simulink model "six_plus_six_AcmsteeringV10_main"  (R2014a)
settings: Solver=FixedStepDiscrete  StartTime=0.0  StopTime=10.0  FixedStep=0.0005  RelTol=1e-3
InitFcn:
  | Veh_Par_wxt
values from neighbouring files (symbols this model uses):
  acc_spdctl = [0 100]    [Veh_Par_wxt.m]
  ag_thr = ecucoder_cal(ag_thr)    [Veh_Par_wxt.m]
  B = 1.8    [Veh_Par_wxt.m]
  bra_em = 100    [Veh_Par_wxt.m]
  bra_pre_gz2 = 100/3    (= 33.3333333333)    [Veh_Par_wxt.m]
  bra_pre_gz34 = 10/3    (= 3.33333333333)    [Veh_Par_wxt.m]
  bra_pre_yd = 10/2    (= 5)    [Veh_Par_wxt.m]
  brakepre_dem_data = [0 1 2 3 4 5 6 7 8 9 10]    [Veh_Par_wxt.m]
  brakeTrq_dem_data = [0 125 251 376 502 627 753 878 1004 1129 1255]    [Veh_Par_wxt.m]
  bratrq_max = 4*1255    (= 5020)    [Veh_Par_wxt.m]
  eff_tran = 0.9    [Veh_Par_wxt.m]
  ESP_switch = ecucoder_cal(ESP_switch)    [Veh_Par_wxt.m]
  G = Mass*g    (= 15696)    [Veh_Par_wxt.m]
  kd1 = ecucoder_cal(kd1)    [Veh_Par_wxt.m]
  kd2 = 0    [Veh_Par_wxt.m]
  ki1 = ecucoder_cal(ki1)    [Veh_Par_wxt.m]
  ki2 = 1    [Veh_Par_wxt.m]
  kp1 = ecucoder_cal(kp1)    [Veh_Par_wxt.m]
  kp2 = 300    [Veh_Par_wxt.m]
  L = L1+L2    (= 2.9)    [Veh_Par_wxt.m]
  premax = 100    [Veh_Par_wxt.m]
  Radius = 0.4572/2    (= 0.2286)    [Veh_Par_wxt.m]
  RC_switch = ecucoder_cal(RC_switch)    [Veh_Par_wxt.m]
  s_opt_yi = 0.15    [Veh_Par_wxt.m]
  s_opt_zhuan = 0.8    [Veh_Par_wxt.m]
  s_opt_zhuan_add = 0.05    [Veh_Par_wxt.m]
  s_opt_zhuan_table = [0.8 0.8 0.3 0.3]    [Veh_Par_wxt.m]
  spd_map_mot = [0 499.85 999.79 1500 2000 2500 3000 3500 4000 4500 4999.8 5999.8]    [Veh_Par_wxt.m]
  spd_spdctl = [0 500]    [Veh_Par_wxt.m]
  speed_thr_park = 5/3.6/Radius*tras_ratio*30/pi    (= 464.143899364)    [Veh_Par_wxt.m]
  TCS_switch = ecucoder_cal(TCS_switch)    [Veh_Par_wxt.m]
  tras_ratio = 8    [Veh_Par_wxt.m]
  trq_map_mot = [70.5 70.012 71.154 65.797 53.917 45.159 38.073 32.685 27.48 17.133 14.949 10.07]    [Veh_Par_wxt.m]
  trqmax_yd = 70.5    [Veh_Par_wxt.m]
  trqmax_zx = 70.5    [Veh_Par_wxt.m]
  trqmaxneg = -70.5    [Veh_Par_wxt.m]
  v_gain = 0.9    [Veh_Par_wxt.m]
  v_table = [0 5 20 100]    [Veh_Par_wxt.m]
  v_thr_park = 5    [Veh_Par_wxt.m]
  zhidong_bianmazhi = [-140000 750000]    [Veh_Par_wxt.m]
  zhidong_down = -140000    [Veh_Par_wxt.m]
  zhidong_up = 750000    [Veh_Par_wxt.m]
  zhidong_youmen = [0 100]    [Veh_Par_wxt.m]
  zhuanxiang_bianmazhi = [-400000 0 400000]    [Veh_Par_wxt.m]
  zhuanxiang_down = -400000    [Veh_Par_wxt.m]
  zhuanxiang_up = 400000    [Veh_Par_wxt.m]
  zhuanxiang_youmen = [-100 0 100]    [Veh_Par_wxt.m]
undefined symbols (not defined in the file or in its folder): ecucoder_acal, guzhang_lf, guzhang_lm, guzhang_lr, guzhang_rf, guzhang_rm, guzhang_rr, myFIS
libraries: simulink x979, ec5744lib x59, fuzblock x2
(part 9 of 27)

== matlab function six_plus_six_AcmsteeringV10_main/MainControl/mode_control/forward/forward/Drive/驱动防滑控制TCS/直行TCS/直行/MATLAB Function7 ==
  data: trq_dem_lf input; trq_dem_lm input; trq_dem_lr input; trq_dem_rf input; trq_dem_rm input; trq_dem_rr input; bra_pre_l input; bra_pre_r input; brake_dem input; flag_lf input; flag_lm input; flag_lr input; trq_out_lf output; trq_out_lm output; flag_rf input; flag_rm input; flag_rr input; trq_out_lr output; trq_out_rf output; trq_out_rm output; trq_out_rr output; trq_pid_lf input; trq_pid_lm input; trq_pid_lr input; trq_pid_rf input; trq_pid_rm input; trq_pid_rr input; brapre_out_l output; brapre_out_r output; mode output
function [trq_out_lf,trq_out_lm,trq_out_lr,trq_out_rf,trq_out_rm,trq_out_rr,brapre_out_l,brapre_out_r,mode] = fcn(trq_dem_lf,trq_dem_lm,trq_dem_lr,trq_dem_rf,trq_dem_rm,trq_dem_rr,bra_pre_l,bra_pre_r,brake_dem,flag_lf,flag_lm,flag_lr,flag_rf,flag_rm,flag_rr,trq_pid_lf,trq_pid_lm,trq_pid_lr,trq_pid_rf,trq_pid_rm,trq_pid_rr)
%#codegen pid模块在外面做，里面进行十六种情况的判断，先看一下效果，不能再修改。
if flag_lf==0 && flag_lm==0 && flag_lr==0 && flag_rf==0 && flag_rm==0 && flag_rr==0 % 0电机滑转===============================================0电机滑转
    trq_out_lf=single(trq_dem_lf);
    trq_out_lm=single(trq_dem_lm);
    trq_out_lr=single(trq_dem_lr);
    trq_out_rf=single(trq_dem_rf);
    trq_out_rm=single(trq_dem_rm);
    trq_out_rr=single(trq_dem_rr);
    brapre_out_l=single(bra_pre_l+brake_dem);
    brapre_out_r=single(bra_pre_r+brake_dem);
    mode=int8(1);
    
    
    
    
    
    
    
    
    
elseif flag_lf==1 && flag_lm==0 && flag_lr==0 && flag_rf==0 && flag_rm==0 && flag_rr==0 %左前轮滑转===================================================1电机滑转
    trq_out_lf=single(trq_pid_lf);
    trq_out_lm=single(trq_dem_lm+(trq_dem_lf-trq_out_lf)/2);
    trq_out_lr=single(trq_dem_lr+(trq_dem_lf-trq_out_lf)/2);
    trq_out_rf=single(trq_dem_rf);
    trq_out_rm=single(trq_dem_rm);
    trq_out_rr=single(trq_dem_rr);
    brapre_out_l=single(bra_pre_l+brake_dem);
    brapre_out_r=single(bra_pre_r+brake_dem);
    mode=int8(2);
elseif flag_lf==0 && flag_lm==1 && flag_lr==0 && flag_rf==0 && flag_rm==0 && flag_rr==0 %左中轮滑转
    trq_out_lm=single(trq_pid_lm);
    trq_out_lf=single(trq_dem_lf+(trq_dem_lm-trq_out_lm)/2);
    trq_out_lr=single(trq_dem_lr+(trq_dem_lm-trq_out_lm)/2);
    trq_out_rf=single(trq_dem_rf);
    trq_out_rm=single(trq_dem_rm);
    trq_out_rr=single(trq_dem_rr);
    brapre_out_l=single(bra_pre_l+brake_dem);
    brapre_out_r=single(bra_pre_r+brake_dem);
    mode=int8(3);
elseif flag_lf==0 && flag_lm==0 && flag_lr==1 && flag_rf==0 && flag_rm==0 && flag_rr==0 %左后轮滑转
    trq_out_lr=single(trq_pid_lr);
    trq_out_lf=single(trq_dem_lf+(trq_dem_lr-trq_out_lr)/2);
    trq_out_lm=single(trq_dem_lm+(trq_dem_lr-trq_out_lr)/2);
    trq_out_rf=single(trq_dem_rf);
    trq_out_rm=single(trq_dem_rm);
    trq_out_rr=single(trq_dem_rr);
    brapre_out_l=single(bra_pre_l+brake_dem);
    brapre_out_r=single(bra_pre_r+brake_dem);
    mode=int8(4);
    
elseif flag_lf==0 && flag_lm==0 && flag_lr==0 && flag_rf==1 && flag_rm==0 && flag_rr==0 %右前轮滑转
    trq_out_rf=single(trq_pid_rf);
    trq_out_rm=single(trq_dem_rm+(trq_dem_rf-trq_out_rf)/2);
    trq_out_rr=single(trq_dem_rr+(trq_dem_rf-trq_out_rf)/2);
    trq_out_lf=single(trq_dem_lf);
    trq_out_lm=single(trq_dem_lm);
    trq_out_lr=single(trq_dem_lr);
    brapre_out_l=single(bra_pre_l+brake_dem);
    brapre_out_r=single(bra_pre_r+brake_dem);
    mode=int8(5);
elseif flag_lf==0 && flag_lm==0 && flag_lr==0 && flag_rf==0 && flag_rm==1 && flag_rr==0 %右中轮滑转
    trq_out_rm=single(trq_pid_rm);
    trq_out_rf=single(trq_dem_rf+(trq_dem_rm-trq_out_rm)/2);
    trq_out_rr=single(trq_dem_rr+(trq_dem_rm-trq_out_rm)/2);
    trq_out_lf=single(trq_dem_lf);
    trq_out_lm=single(trq_dem_lm);
    trq_out_lr=single(trq_dem_lr);
    brapre_out_l=single(bra_pre_l+brake_dem);
    brapre_out_r=single(bra_pre_r+brake_dem);
    mode=int8(6);
elseif flag_lf==0 && flag_lm==0 && flag_lr==0 && flag_rf==0 && flag_rm==0 && flag_rr==1 %右后轮滑转
    trq_out_rr=single(trq_pid_rr);
    trq_out_rf=single(trq_dem_rf+(trq_dem_rr-trq_out_rr)/2);
    trq_out_rm=single(trq_dem_rm+(trq_dem_rr-trq_out_rr)/2);
    trq_out_lf=single(trq_dem_lf);
    trq_out_lm=single(trq_dem_lm);
    trq_out_lr=single(trq_dem_lr);
    brapre_out_l=single(bra_pre_l+brake_dem);
    brapre_out_r=single(bra_pre_r+brake_dem);
    mode=int8(7);
    
    
    
    
    
    
    
    
    
    
elseif flag_lf==1 && flag_lm==1 && flag_lr==0 && flag_rf==0 && flag_rm==0 && flag_rr==0 %左前-左中 轮滑转===================================================2电机滑转    左侧
    trq_out_lf=single(trq_pid_lf);
    trq_out_lm=single(trq_pid_lm);
    trq_out_lr=single(trq_dem_lr+(trq_dem_lf-trq_out_lf)+(trq_dem_lm-trq_out_lm));
    trq_out_rf=single(trq_dem_rf);
    trq_out_rm=single(trq_dem_rm);
    trq_out_rr=single(trq_dem_rr);
    brapre_out_l=single(bra_pre_l+brake_dem);
    brapre_out_r=single(bra_pre_r+brake_dem);
    mode=int8(8);
elseif flag_lf==1 && flag_lm==0 && flag_lr==1 && flag_rf==0 && flag_rm==0 && flag_rr==0 %左前-左后 轮滑转
    trq_out_lf=single(trq_pid_lf);
    trq_out_lr=single(trq_pid_lr);
    trq_out_lm=single(trq_dem_lm+(trq_dem_lf-trq_out_lf)+(trq_dem_lr-trq_out_lr));
    trq_out_rf=single(trq_dem_rf);
    trq_out_rm=single(trq_dem_rm);
    trq_out_rr=single(trq_dem_rr);
    brapre_out_l=single(bra_pre_l+brake_dem);
    brapre_out_r=single(bra_pre_r+brake_dem);
    mode=int8(9);
elseif flag_lf==0 && flag_lm==1 && flag_lr==1 && flag_rf==0 && flag_rm==0 && flag_rr==0 %左中-左后 轮滑转
    trq_out_lm=single(trq_pid_lm);
    trq_out_lr=single(trq_pid_lr);
    trq_out_lf=single(trq_dem_lf+(trq_dem_lm-trq_out_lm)+(trq_dem_lr-trq_out_lr));
    trq_out_rf=single(trq_dem_rf);
    trq_out_rm=single(trq_dem_rm);
    trq_out_rr=single(trq_dem_rr);
    brapre_out_l=single(bra_pre_l+brake_dem);
    brapre_out_r=single(bra_pre_r+brake_dem);
    mode=int8(10);
    
elseif flag_lf==0 && flag_lm==0 && flag_lr==0 && flag_rf==1 && flag_rm==1 && flag_rr==0 %右前-右中 轮滑转                        右侧
    trq_out_rf=single(trq_pid_rf);
    trq_out_rm=single(trq_pid_rm);
    trq_out_rr=single(trq_dem_rr+(trq_dem_rf-trq_out_rf)+(trq_dem_rm-trq_out_rm));
    trq_out_lf=single(trq_dem_lf);
    trq_out_lm=single(trq_dem_lm);
    trq_out_lr=single(trq_dem_lr);
    brapre_out_l=single(bra_pre_l+brake_dem);
    brapre_out_r=single(bra_pre_r+brake_dem);
    mode=int8(11);
elseif flag_lf==0 && flag_lm==0 && flag_lr==0 && flag_rf==1 && flag_rm==0 && flag_rr==1 %右前-右后 轮滑转
    trq_out_rf=single(trq_pid_rf);
    trq_out_rr=single(trq_pid_rr);
    trq_out_rm=single(trq_dem_rm+(trq_dem_rf-trq_out_rf)+(trq_dem_rr-trq_out_rr));
    trq_out_lf=single(trq_dem_lf);
    trq_out_lm=single(trq_dem_lm);
    trq_out_lr=single(trq_dem_lr);
    brapre_out_l=single(bra_pre_l+brake_dem);
    brapre_out_r=single(bra_pre_r+brake_dem);
    mode=int8(12);
elseif flag_lf==0 && flag_lm==0 && flag_lr==0 && flag_rf==0 && flag_rm==1 && flag_rr==1 %右中-右后 轮滑转
    trq_out_rm=single(trq_pid_rm);
    trq_out_rr=single(trq_pid_rr);
    trq_out_rf=single(trq_dem_rf+(trq_dem_rm-trq_out_rm)+(trq_dem_rr-trq_out_rr));
    trq_out_lf=single(trq_dem_lf);
    trq_out_lm=single(trq_dem_lm);
    trq_out_lr=single(trq_dem_lr);
    brapre_out_l=single(bra_pre_l+brake_dem);
    brapre_out_r=single(bra_pre_r+brake_dem);
    mode=int8(13);
    
elseif flag_lf==1 && flag_lm==0 && flag_lr==0 && flag_rf==1 && flag_rm==0 && flag_rr==0 %左前-右前 轮滑转                 对侧
    trq_out_lf=single(trq_pid_lf);
    trq_out_lm=single(trq_dem_lm+(trq_dem_lf-trq_out_lf)/2);
    trq_out_lr=single(trq_dem_lr+(trq_dem_lf-trq_out_lf)/2);
    trq_out_rf=single(trq_pid_rf);
    trq_out_rm=single(trq_dem_rm+(trq_dem_rf-trq_out_rf)/2);
    trq_out_rr=single(trq_dem_rr+(trq_dem_rf-trq_out_rf)/2);
    brapre_out_l=single(bra_pre_l+brake_dem);
    brapre_out_r=single(bra_pre_r+brake_dem);
    mode=int8(14);
elseif flag_lf==1 && flag_lm==0 && flag_lr==0 && flag_rf==0 && flag_rm==1 && flag_rr==0 %左前-右中 轮滑转
    trq_out_lf=single(trq_pid_lf);
    trq_out_lm=single(trq_dem_lm+(trq_dem_lf-trq_out_lf)/2);
    trq_out_lr=single(trq_dem_lr+(trq_dem_lf-trq_out_lf)/2);
    trq_out_rm=single(trq_pid_rm);
    trq_out_rf=single(trq_dem_rf+(trq_dem_rm-trq_out_rm)/2);
    trq_out_rr=single(trq_dem_rr+(trq_dem_rm-trq_out_rm)/2);
    brapre_out_l=single(bra_pre_l+brake_dem);
    brapre_out_r=single(bra_pre_r+brake_dem);
    mode=int8(15);
elseif flag_lf==1 && flag_lm==0 && flag_lr==0 && flag_rf==0 && flag_rm==0 && flag_rr==1 %左前-右后 轮滑转
    trq_out_lf=single(trq_pid_lf);
    trq_out_lm=single(trq_dem_lm+(trq_dem_lf-trq_out_lf)/2);
    trq_out_lr=single(trq_dem_lr+(trq_dem_lf-trq_out_lf)/2);
    trq_out_rr=single(trq_pid_rr);
    trq_out_rf=single(trq_dem_rf+(trq_dem_rr-trq_out_rr)/2);
    trq_out_rm=single(trq_dem_rm+(trq_dem_rr-trq_out_rr)/2);
    brapre_out_l=single(bra_pre_l+brake_dem);
    brapre_out_r=single(bra_pre_r+brake_dem);
    mode=int8(16);
    
elseif flag_lf==0 && flag_lm==1 && flag_lr==0 && flag_rf==1 && flag_rm==0 && flag_rr==0 %左中-右前 轮滑转                 对侧
    trq_out_lm=single(trq_pid_lm);
    trq_out_lf=single(trq_dem_lf+(trq_dem_lm-trq_out_lm)/2);
    trq_out_lr=single(trq_dem_lr+(trq_dem_lm-trq_out_lm)/2);
    trq_out_rf=single(trq_pid_rf);
    trq_out_rm=single(trq_dem_rm+(trq_dem_rf-trq_out_rf)/2);
    trq_out_rr=single(trq_dem_rr+(trq_dem_rf-trq_out_rf)/2);
    brapre_out_l=single(bra_pre_l+brake_dem);
    brapre_out_r=single(bra_pre_r+brake_dem);
    mode=int8(17);
elseif flag_lf==0 && flag_lm==1 && flag_lr==0 && flag_rf==0 && flag_rm==1 && flag_rr==0 %左中-右中 轮滑转
    trq_out_lm=single(trq_pid_lm);
    trq_out_lf=single(trq_dem_lf+(trq_dem_lm-trq_out_lm)/2);
    trq_out_lr=single(trq_dem_lr+(trq_dem_lm-trq_out_lm)/2);
    trq_out_rm=single(trq_pid_rm);
    trq_out_rf=single(trq_dem_rf+(trq_dem_rm-trq_out_rm)/2);
    trq_out_rr=single(trq_dem_rr+(trq_dem_rm-trq_out_rm)/2);
    brapre_out_l=single(bra_pre_l+brake_dem);
    brapre_out_r=single(bra_pre_r+brake_dem);
    mode=int8(18);
elseif flag_lf==0 && flag_lm==1 && flag_lr==0 && flag_rf==0 && flag_rm==0 && flag_rr==1 %左中-右后 轮滑转
    trq_out_lm=single(trq_pid_lm);
    trq_out_lf=single(trq_dem_lf+(trq_dem_lm-trq_out_lm)/2);
    trq_out_lr=single(trq_dem_lr+(trq_dem_lm-trq_out_lm)/2);
    trq_out_rr=single(trq_pid_rr);
    trq_out_rf=single(trq_dem_rf+(trq_dem_rr-trq_out_rr)/2);
    trq_out_rm=single(trq_dem_rm+(trq_dem_rr-trq_out_rr)/2);
    brapre_out_l=single(bra_pre_l+brake_dem);
    brapre_out_r=single(bra_pre_r+brake_dem);
    mode=int8(19);
elseif flag_lf==0 && flag_lm==0 && flag_lr==1 && flag_rf==1 && flag_rm==0 && flag_rr==0 %左后-右前 轮滑转                 对侧
    trq_out_lr=single(trq_pid_lr);
    trq_out_lf=single(trq_dem_lf+(trq_dem_lr-trq_out_lr)/2);
    trq_out_lm=single(trq_dem_lm+(trq_dem_lr-trq_out_lr)/2);
    trq_out_rf=single(trq_pid_rf);
    trq_out_rm=single(trq_dem_rm+(trq_dem_rf-trq_out_rf)/2);
    trq_out_rr=single(trq_dem_rr+(trq_dem_rf-trq_out_rf)/2);
    brapre_out_l=single(bra_pre_l+brake_dem);
    brapre_out_r=single(bra_pre_r+brake_dem);
    mode=int8(20);
elseif flag_lf==0 && flag_lm==0 && flag_lr==1 && flag_rf==0 && flag_rm==1 && flag_rr==0 %左后-右中 轮滑转
    trq_out_lr=single(trq_pid_lr);
    trq_out_lf=single(trq_dem_lf+(trq_dem_lr-trq_out_lr)/2);
    trq_out_lm=single(trq_dem_lm+(trq_dem_lr-trq_out_lr)/2);
    trq_out_rm=single(trq_pid_rm);
    trq_out_rf=single(trq_dem_rf+(trq_dem_rm-trq_out_rm)/2);
    trq_out_rr=single(trq_dem_rr+(trq_dem_rm-trq_out_rm)/2);
    brapre_out_l=single(bra_pre_l+brake_dem);
    brapre_out_r=single(bra_pre_r+brake_dem);
    mode=int8(21);
elseif flag_lf==0 && flag_lm==0 && flag_lr==1 && flag_rf==0 && flag_rm==0 && flag_rr==1 %左后-右后 轮滑转
    trq_out_lr=single(trq_pid_lr);
    trq_out_lf=single(trq_dem_lf+(trq_dem_lr-trq_out_lr)/2);
    trq_out_lm=single(trq_dem_lm+(trq_dem_lr-trq_out_lr)/2);
    trq_out_rr=single(trq_pid_rr);
    trq_out_rf=single(trq_dem_rf+(trq_dem_rr-trq_out_rr)/2);
    trq_out_rm=single(trq_dem_rm+(trq_dem_rr-trq_out_rr)/2);
    brapre_out_l=single(bra_pre_l+brake_dem);
    brapre_out_r=single(bra_pre_r+brake_dem);
    mode=int8(22);
    
    
    
    
    
    
    
    
    
    
    
    
    
    
    
    
    
    
    
    
    
    
elseif flag_lf==1 && flag_lm==1 && flag_lr==1 && flag_rf==0 && flag_rm==0 && flag_rr==0 %左前-左中-左后 轮滑转===================================================3电机滑转    左侧
    trq_out_lf=single(trq_pid_lf);
    trq_out_lm=single(trq_pid_lm);
    trq_out_lr=single(trq_pid_lr);
    trq_out_rf=single(trq_dem_rf-((trq_dem_lf-trq_out_lf)+(trq_dem_lm-trq_out_lm)+(trq_dem_lr-trq_out_lr))/3);
    trq_out_rm=single(trq_dem_rm-((trq_dem_lf-trq_out_lf)+(trq_dem_lm-trq_out_lm)+(trq_dem_lr-trq_out_lr))/3);
    trq_out_rr=single(trq_dem_rr-((trq_dem_lf-trq_out_lf)+(trq_dem_lm-trq_out_lm)+(trq_dem_lr-trq_out_lr))/3);
    brapre_out_l=single(bra_pre_l+brake_dem);
    brapre_out_r=single(bra_pre_r+brake_dem);
    mode=int8(23);
elseif flag_lf==0 && flag_lm==0 && flag_lr==0 && flag_rf==1 && flag_rm==1 && flag_rr==1 %右前-右中-右后 轮滑转                      右侧
    trq_out_rf=single(trq_pid_rf);
    trq_out_rm=single(trq_pid_rm);
    trq_out_rr=single(trq_pid_rr);
    trq_out_lf=single(trq_dem_lf-((trq_dem_rf-trq_out_rf)+(trq_dem_rm-trq_out_rm)+(trq_dem_rr-trq_out_rr))/3);
    trq_out_lm=single(trq_dem_lm-((trq_dem_rf-trq_out_rf)+(trq_dem_rm-trq_out_rm)+(trq_dem_rr-trq_out_rr))/3);
    trq_out_lr=single(trq_dem_lr-((trq_dem_rf-trq_out_rf)+(trq_dem_rm-trq_out_rm)+(trq_dem_rr-trq_out_rr))/3);
    brapre_out_l=single(bra_pre_l+brake_dem);
    brapre_out_r=single(bra_pre_r+brake_dem);
    mode=int8(24);
    
elseif flag_lf==1 && flag_lm==1 && flag_lr==0 && flag_rf==1 && flag_rm==0 && flag_rr==0 %左前-左中-右前 轮滑转
    trq_out_lf=single(trq_pid_lf);
    trq_out_lm=single(trq_pid_lm);
    trq_out_lr=single(trq_dem_lr+(trq_dem_lf-trq_out_lf)+(trq_dem_lm-trq_out_lm));
    trq_out_rf=single(trq_pid_rf);
    trq_out_rm=single(trq_dem_rm+(trq_dem_rf-trq_out_rf)/2);
    trq_out_rr=single(trq_dem_rr+(trq_dem_rf-trq_out_rf)/2);
    brapre_out_l=single(bra_pre_l+brake_dem);
    brapre_out_r=single(bra_pre_r+brake_dem);
    mode=int8(25);
elseif flag_lf==1 && flag_lm==1 && flag_lr==0 && flag_rf==0 && flag_rm==1 && flag_rr==0 %左前-左中-右中 轮滑转
    trq_out_lf=single(trq_pid_lf);
    trq_out_lm=single(trq_pid_lm);
    trq_out_lr=single(trq_dem_lr+(trq_dem_lf-trq_out_lf)+(trq_dem_lm-trq_out_lm));
    trq_out_rm=single(trq_pid_rm);
    trq_out_rf=single(trq_dem_rf+(trq_dem_rm-trq_out_rm)/2);
    trq_out_rr=single(trq_dem_rr+(trq_dem_rm-trq_out_rm)/2);
    brapre_out_l=single(bra_pre_l+brake_dem);
    brapre_out_r=single(bra_pre_r+brake_dem);
    mode=int8(26);
elseif flag_lf==1 && flag_lm==1 && flag_lr==0 && flag_rf==0 && flag_rm==0 && flag_rr==1 %左前-左中-右后 轮滑转
    trq_out_lf=single(trq_pid_lf);
    trq_out_lm=single(trq_pid_lm);
    trq_out_lr=single(trq_dem_lr+(trq_dem_lf-trq_out_lf)+(trq_dem_lm-trq_out_lm));
    trq_out_rr=single(trq_pid_rr);
    trq_out_rf=single(trq_dem_rf+(trq_dem_rr-trq_out_rr)/2);
    trq_out_rm=single(trq_dem_rm+(trq_dem_rr-trq_out_rr)/2);
    brapre_out_l=single(bra_pre_l+brake_dem);
    brapre_out_r=single(bra_pre_r+brake_dem);
    mode=int8(27);
    
elseif flag_lf==1 && flag_lm==0 && flag_lr==1 && flag_rf==1 && flag_rm==0 && flag_rr==0 %左前-左后-右前 轮滑转
    trq_out_lf=single(trq_pid_lf);
    trq_out_lr=single(trq_pid_lr);
    trq_out_lm=single(trq_dem_lm+(trq_dem_lf-trq_out_lf)+(trq_dem_lr-trq_out_lr));
    trq_out_rf=single(trq_pid_rf);
    trq_out_rm=single(trq_dem_rm+(trq_dem_rf-trq_out_rf)/2);
    trq_out_rr=single(trq_dem_rr+(trq_dem_rf-trq_out_rf)/2);
    brapre_out_l=single(bra_pre_l+brake_dem);
    brapre_out_r=single(bra_pre_r+brake_dem);
    mode=int8(28);
elseif flag_lf==1 && flag_lm==0 && flag_lr==1 && flag_rf==0 && flag_rm==1 && flag_rr==0 %左前-左后-右中 轮滑转
    trq_out_lf=single(trq_pid_lf);
    trq_out_lr=single(trq_pid_lr);
    trq_out_lm=single(trq_dem_lm+(trq_dem_lf-trq_out_lf)+(trq_dem_lr-trq_out_lr));
    trq_out_rm=single(trq_pid_rm);
    trq_out_rf=single(trq_dem_rf+(trq_dem_rm-trq_out_rm)/2);
    trq_out_rr=single(trq_dem_rr+(trq_dem_rm-trq_out_rm)/2);
    brapre_out_l=single(bra_pre_l+brake_dem);
    brapre_out_r=single(bra_pre_r+brake_dem);
    mode=int8(29);
elseif flag_lf==1 && flag_lm==0 && flag_lr==1 && flag_rf==0 && flag_rm==0 && flag_rr==1 %左前-左后-右后 轮滑转
    trq_out_lf=single(trq_pid_lf);
    trq_out_lr=single(trq_pid_lr);
    trq_out_lm=single(trq_dem_lm+(trq_dem_lf-trq_out_lf)+(trq_dem_lr-trq_out_lr));
    trq_out_rr=single(trq_pid_rr);
    trq_out_rf=single(trq_dem_rf+(trq_dem_rr-trq_out_rr)/2);
    trq_out_rm=single(trq_dem_rm+(trq_dem_rr-trq_out_rr)/2);
    brapre_out_l=single(bra_pre_l+brake_dem);
    brapre_out_r=single(bra_pre_r+brake_dem);
    mode=int8(30);
    
elseif flag_lf==0 && flag_lm==1 && flag_lr==1 && flag_rf==1 && flag_rm==0 && flag_rr==0 %左中-左后-右前 轮滑转
    trq_out_lm=single(trq_pid_lm);
    trq_out_lr=single(trq_pid_lr);
    trq_out_lf=single(trq_dem_lf+(trq_dem_lm-trq_out_lm)+(trq_dem_lr-trq_out_lr));
    trq_out_rf=single(trq_pid_rf);
    trq_out_rm=single(trq_dem_rm+(trq_dem_rf-trq_out_rf)/2);
    trq_out_rr=single(trq_dem_rr+(trq_dem_rf-trq_out_rf)/2);
    brapre_out_l=single(bra_pre_l+brake_dem);
    brapre_out_r=single(bra_pre_r+brake_dem);
    mode=int8(31);
elseif flag_lf==0 && flag_lm==1 && flag_lr==1 && flag_rf==0 && flag_rm==1 && flag_rr==0 %左中-左后-右中 轮滑转
    trq_out_lm=single(trq_pid_lm);
    trq_out_lr=single(trq_pid_lr);
    trq_out_lf=single(trq_dem_lf+(trq_dem_lm-trq_out_lm)+(trq_dem_lr-trq_out_lr));
    trq_out_rm=single(trq_pid_rm);
    trq_out_rf=single(trq_dem_rf+(trq_dem_rm-trq_out_rm)/2);
    trq_out_rr=single(trq_dem_rr+(trq_dem_rm-trq_out_rm)/2);
    brapre_out_l=single(bra_pre_l+brake_dem);
    brapre_out_r=single(bra_pre_r+brake_dem);
    mode=int8(32);
elseif flag_lf==0 && flag_lm==1 && flag_lr==1 && flag_rf==0 && flag_rm==0 && flag_rr==1 %左中-左后-右后 轮滑转
    trq_out_lm=single(trq_pid_lm);
    trq_out_lr=single(trq_pid_lr);
    trq_out_lf=single(trq_dem_lf+(trq_dem_lm-trq_out_lm)+(trq_dem_lr-trq_out_lr));
    trq_out_rr=single(trq_pid_rr);
    trq_out_rf=single(trq_dem_rf+(trq_dem_rr-trq_out_rr)/2);
    trq_out_rm=single(trq_dem_rm+(trq_dem_rr-trq_out_rr)/2);
    brapre_out_l=single(bra_pre_l+brake_dem);
    brapre_out_r=single(bra_pre_r+brake_dem);
    mode=int8(33);
    
elseif flag_lf==1 && flag_lm==0 && flag_lr==0 && flag_rf==1 && flag_rm==1 && flag_rr==0 %右前-右中-左前 轮滑转
    trq_out_rf=single(trq_pid_rf);
    trq_out_rm=single(trq_pid_rm);
    trq_out_rr=single(trq_dem_rr+(trq_dem_rf-trq_out_rf)+(trq_dem_rm-trq_out_rm));
    trq_out_lf=single(trq_pid_lf);
    trq_out_lm=single(trq_dem_lm+(trq_dem_lf-trq_out_lf)/2);
    trq_out_lr=single(trq_dem_lr+(trq_dem_lf-trq_out_lf)/2);
    brapre_out_l=single(bra_pre_l+brake_dem);
    brapre_out_r=single(bra_pre_r+brake_dem);
    mode=int8(34);
elseif flag_lf==0 && flag_lm==1 && flag_lr==0 && flag_rf==1 && flag_rm==1 && flag_rr==0 %右前-右中-左中 轮滑转
    trq_out_rf=single(trq_pid_rf);
    trq_out_rm=single(trq_pid_rm);
    trq_out_rr=single(trq_dem_rr+(trq_dem_rf-trq_out_rf)+(trq_dem_rm-trq_out_rm));
    trq_out_lm=single(trq_pid_lm);
    trq_out_lf=single(trq_dem_lf+(trq_dem_lm-trq_out_lm)/2);
    trq_out_lr=single(trq_dem_lr+(trq_dem_lm-trq_out_lm)/2);
    brapre_out_l=single(bra_pre_l+brake_dem);
    brapre_out_r=single(bra_pre_r+brake_dem);
    mode=int8(35);
elseif flag_lf==0 && flag_lm==0 && flag_lr==1 && flag_rf==1 && flag_rm==1 && flag_rr==0 %右前-右中-左后 轮滑转
    trq_out_rf=single(trq_pid_rf);
    trq_out_rm=single(trq_pid_rm);
    trq_out_rr=single(trq_dem_rr+(trq_dem_rf-trq_out_rf)+(trq_dem_rm-trq_out_rm));
    trq_out_lr=single(trq_pid_lr);
    trq_out_lf=single(trq_dem_lf+(trq_dem_lr-trq_out_lr)/2);
    trq_out_lm=single(trq_dem_lm+(trq_dem_lr-trq_out_lr)/2);
    brapre_out_l=single(bra_pre_l+brake_dem);
    brapre_out_r=single(bra_pre_r+brake_dem);
    mode=int8(36);
    
elseif flag_lf==1 && flag_lm==0 && flag_lr==0 && flag_rf==1 && flag_rm==0 && flag_rr==1 %右前-右后-左前 轮滑转
    trq_out_rf=single(trq_pid_rf);
    trq_out_rr=single(trq_pid_rr);
    trq_out_rm=single(trq_dem_rm+(trq_dem_rf-trq_out_rf)+(trq_dem_rr-trq_out_rr));
    trq_out_lf=single(trq_pid_lf);
    trq_out_lm=single(trq_dem_lm+(trq_dem_lf-trq_out_lf)/2);
    trq_out_lr=single(trq_dem_lr+(trq_dem_lf-trq_out_lf)/2);
    brapre_out_l=single(bra_pre_l+brake_dem);
    brapre_out_r=single(bra_pre_r+brake_dem);
    mode=int8(37);
elseif flag_lf==0 && flag_lm==1 && flag_lr==0 && flag_rf==1 && flag_rm==0 && flag_rr==1 %右前-右后-左中 轮滑转
    trq_out_rf=single(trq_pid_rf);
    trq_out_rr=single(trq_pid_rr);
    trq_out_rm=single(trq_dem_rm+(trq_dem_rf-trq_out_rf)+(trq_dem_rr-trq_out_rr));
    trq_out_lm=single(trq_pid_lm);
    trq_out_lf=single(trq_dem_lf+(trq_dem_lm-trq_out_lm)/2);
    trq_out_lr=single(trq_dem_lr+(trq_dem_lm-trq_out_lm)/2);
    brapre_out_l=single(bra_pre_l+brake_dem);
    brapre_out_r=single(bra_pre_r+brake_dem);
    mode=int8(38);
elseif flag_lf==0 && flag_lm==0 && flag_lr==1 && flag_rf==1 && flag_rm==0 && flag_rr==1 %右前-右后-左后 轮滑转
    trq_out_rf=single(trq_pid_rf);
    trq_out_rr=single(trq_pid_rr);
    trq_out_rm=single(trq_dem_rm+(trq_dem_rf-trq_out_rf)+(trq_dem_rr-trq_out_rr));
    trq_out_lr=single(trq_pid_lr);
    trq_out_lf=single(trq_dem_lf+(trq_dem_lr-trq_out_lr)/2);
    trq_out_lm=single(trq_dem_lm+(trq_dem_lr-trq_out_lr)/2);
    brapre_out_l=single(bra_pre_l+brake_dem);
    brapre_out_r=single(bra_pre_r+brake_dem);
    mode=int8(39);
    
elseif flag_lf==1 && flag_lm==0 && flag_lr==0 && flag_rf==0 && flag_rm==1 && flag_rr==1 %右中-右后-左前 轮滑转
    trq_out_rm=single(trq_pid_rm);
    trq_out_rr=single(trq_pid_rr);
    trq_out_rf=single(trq_dem_rf+(trq_dem_rm-trq_out_rm)+(trq_dem_rr-trq_out_rr));
    trq_out_lf=single(trq_pid_lf);
    trq_out_lm=single(trq_dem_lm+(trq_dem_lf-trq_out_lf)/2);
    trq_out_lr=single(trq_dem_lr+(trq_dem_lf-trq_out_lf)/2);
    brapre_out_l=single(bra_pre_l+brake_dem);
    brapre_out_r=single(bra_pre_r+brake_dem);
    mode=int8(40);
elseif flag_lf==0 && flag_lm==1 && flag_lr==0 && flag_rf==0 && flag_rm==1 && flag_rr==1 %右中-右后-左中 轮滑转
    trq_out_rm=single(trq_pid_rm);
    trq_out_rr=single(trq_pid_rr);
    trq_out_rf=single(trq_dem_rf+(trq_dem_rm-trq_out_rm)+(trq_dem_rr-trq_out_rr));
    trq_out_lm=single(trq_pid_lm);
    trq_out_lf=single(trq_dem_lf+(trq_dem_lm-trq_out_lm)/2);
    trq_out_lr=single(trq_dem_lr+(trq_dem_lm-trq_out_lm)/2);
    brapre_out_l=single(bra_pre_l+brake_dem);
    brapre_out_r=single(bra_pre_r+brake_dem);
    mode=int8(41);
elseif flag_lf==0 && flag_lm==0 && flag_lr==1 && flag_rf==0 && flag_rm==1 && flag_rr==1 %右中-右后-左后 轮滑转
    trq_out_rm=single(trq_pid_rm);
    trq_out_rr=single(trq_pid_rr);
    trq_out_rf=single(trq_dem_rf+(trq_dem_rm-trq_out_rm)+(trq_dem_rr-trq_out_rr));
    trq_out_lr=single(trq_pid_lr);
    trq_out_lf=single(trq_dem_lf+(trq_dem_lr-trq_out_lr)/2);
    trq_out_lm=single(trq_dem_lm+(trq_dem_lr-trq_out_lr)/2);
    brapre_out_l=single(bra_pre_l+brake_dem);
    brapre_out_r=single(bra_pre_r+brake_dem);
    mode=int8(42);
    
    
    
    
    
    
    
    
    
    
    
    
    
    
    
    
    
    
    
    
    
elseif flag_lf==1 && flag_lm==1 && flag_lr==1 && flag_rf==1 && flag_rm==0 && flag_rr==0 %左前-左中-左后 右前 轮滑转===================================================4电机滑转
    trq_out_lf=single(trq_pid_lf);
    trq_out_lm=single(trq_pid_lm);
    trq_out_lr=single(trq_pid_lr);
    trq_out_rf=single(trq_pid_rf);
    trq_out_rm=single(trq_dem_rm-((trq_dem_lf-trq_out_lf)+(trq_dem_lm-trq_out_lm)+(trq_dem_lr-trq_out_lr)-(trq_dem_rf-trq_out_rf))/2);
    trq_out_rr=single(trq_dem_rr-((trq_dem_lf-trq_out_lf)+(trq_dem_lm-trq_out_lm)+(trq_dem_lr-trq_out_lr)-(trq_dem_rf-trq_out_rf))/2);
    brapre_out_l=single(bra_pre_l+brake_dem);
    brapre_out_r=single(bra_pre_r+brake_dem);
    mode=int8(43);
elseif flag_lf==1 && flag_lm==1 && flag_lr==1 && flag_rf==0 && flag_rm==1 && flag_rr==0 %左前-左中-左后 右中 轮滑转
    trq_out_lf=single(trq_pid_lf);
    trq_out_lm=single(trq_pid_lm);
    trq_out_lr=single(trq_pid_lr);
    trq_out_rm=single(trq_pid_rm);
    trq_out_rf=single(trq_dem_rf-((trq_dem_lf-trq_out_lf)+(trq_dem_lm-trq_out_lm)+(trq_dem_lr-trq_out_lr)-(trq_dem_rm-trq_out_rm))/2);
    trq_out_rr=single(trq_dem_rr-((trq_dem_lf-trq_out_lf)+(trq_dem_lm-trq_out_lm)+(trq_dem_lr-trq_out_lr)-(trq_dem_rm-trq_out_rm))/2);
    brapre_out_l=single(bra_pre_l+brake_dem);
    brapre_out_r=single(bra_pre_r+brake_dem);
    mode=int8(44);
elseif flag_lf==1 && flag_lm==1 && flag_lr==1 && flag_rf==0 && flag_rm==0 && flag_rr==1 %左前-左中-左后 右后 轮滑转
    trq_out_lf=single(trq_pid_lf);
    trq_out_lm=single(trq_pid_lm);
    trq_out_lr=single(trq_pid_lr);
    trq_out_rr=single(trq_pid_rr);
    trq_out_rf=single(trq_dem_rf-((trq_dem_lf-trq_out_lf)+(trq_dem_lm-trq_out_lm)+(trq_dem_lr-trq_out_lr)-(trq_dem_rr-trq_out_rr))/2);
    trq_out_rm=single(trq_dem_rm-((trq_dem_lf-trq_out_lf)+(trq_dem_lm-trq_out_lm)+(trq_dem_lr-trq_out_lr)-(trq_dem_rr-trq_out_rr))/2);
    brapre_out_l=single(bra_pre_l+brake_dem);
    brapre_out_r=single(bra_pre_r+brake_dem);
    mode=int8(45);
    
elseif flag_lf==1 && flag_lm==0 && flag_lr==0 && flag_rf==1 && flag_rm==1 && flag_rr==1 %右前-右中-右后 左前 轮滑转
    trq_out_rf=single(trq_pid_rf);
    trq_out_rm=single(trq_pid_rm);
    trq_out_rr=single(trq_pid_rr);
    trq_out_lf=single(trq_pid_lf);
    trq_out_lm=single(trq_dem_lm-((trq_dem_rf-trq_out_rf)+(trq_dem_rm-trq_out_rm)+(trq_dem_rr-trq_out_rr)-(trq_dem_lf-trq_out_lf))/2);
    trq_out_lr=single(trq_dem_lr-((trq_dem_rf-trq_out_rf)+(trq_dem_rm-trq_out_rm)+(trq_dem_rr-trq_out_rr)-(trq_dem_lf-trq_out_lf))/2);
    brapre_out_l=single(bra_pre_l+brake_dem);
    brapre_out_r=single(bra_pre_r+brake_dem);
    mode=int8(46);
elseif flag_lf==0 && flag_lm==1 && flag_lr==0 && flag_rf==1 && flag_rm==1 && flag_rr==1 %右前-右中-右后 左中 轮滑转
    trq_out_rf=single(trq_pid_rf);
    trq_out_rm=single(trq_pid_rm);
    trq_out_rr=single(trq_pid_rr);
    trq_out_lm=single(trq_pid_lm);
    trq_out_lf=single(trq_dem_lf-((trq_dem_rf-trq_out_rf)+(trq_dem_rm-trq_out_rm)+(trq_dem_rr-trq_out_rr)-(trq_dem_lm-trq_out_lm))/2);
    trq_out_lr=single(trq_dem_lr-((trq_dem_rf-trq_out_rf)+(trq_dem_rm-trq_out_rm)+(trq_dem_rr-trq_out_rr)-(trq_dem_lm-trq_out_lm))/2);
    brapre_out_l=single(bra_pre_l+brake_dem);
    brapre_out_r=single(bra_pre_r+brake_dem);
    mode=int8(47);
elseif flag_lf==0 && flag_lm==0 && flag_lr==1 && flag_rf==1 && flag_rm==1 && flag_rr==1 %右前-右中-右后 左后 轮滑转
    trq_out_rf=single(trq_pid_rf);
    trq_out_rm=single(trq_pid_rm);
    trq_out_rr=single(trq_pid_rr);
    trq_out_lr=single(trq_pid_lr);
    trq_out_lf=single(trq_dem_lf-((trq_dem_rf-trq_out_rf)+(trq_dem_rm-trq_out_rm)+(trq_dem_rr-trq_out_rr)-(trq_dem_lr-trq_out_lr))/2);
    trq_out_lm=single(trq_dem_lm-((trq_dem_rf-trq_out_rf)+(trq_dem_rm-trq_out_rm)+(trq_dem_rr-trq_out_rr)-(trq_dem_lr-trq_out_lr))/2);
    brapre_out_l=single(bra_pre_l+brake_dem);
    brapre_out_r=single(bra_pre_r+brake_dem);
    mode=int8(48);
    
elseif flag_lf==1 && flag_lm==1 && flag_lr==0 && flag_rf==1 && flag_rm==1 && flag_rr==0 %左前-左中 右前-右中 轮滑转
    trq_out_lf=single(trq_pid_lf);
    trq_out_lm=single(trq_pid_lm);
    trq_out_lr=single(trq_dem_lr+(trq_dem_lf-trq_out_lf)+(trq_dem_lm-trq_out_lm));
    trq_out_rf=single(trq_pid_rf);
    trq_out_rm=single(trq_pid_rm);
    trq_out_rr=single(trq_dem_rr+(trq_dem_rf-trq_out_rf)+(trq_dem_rm-trq_out_rm));
    brapre_out_l=single(bra_pre_l+brake_dem);
    brapre_out_r=single(bra_pre_r+brake_dem);
    mode=int8(49);
elseif flag_lf==1 && flag_lm==1 && flag_lr==0 && flag_rf==1 && flag_rm==0 && flag_rr==1 %左前-左中 右前-右后 轮滑转
    trq_out_lf=single(trq_pid_lf);
    trq_out_lm=single(trq_pid_lm);
    trq_out_lr=single(trq_dem_lr+(trq_dem_lf-trq_out_lf)+(trq_dem_lm-trq_out_lm));
    trq_out_rf=single(trq_pid_rf);
    trq_out_rr=single(trq_pid_rr);
    trq_out_rm=single(trq_dem_rm+(trq_dem_rf-trq_out_rf)+(trq_dem_rr-trq_out_rr));
    brapre_out_l=single(bra_pre_l+brake_dem);
    brapre_out_r=single(bra_pre_r+brake_dem);
    mode=int8(50);
elseif flag_lf==1 && flag_lm==1 && flag_lr==0 && flag_rf==0 && flag_rm==1 && flag_rr==1 %左前-左中 右中-右后 轮滑转
    trq_out_lf=single(trq_pid_lf);
    trq_out_lm=single(trq_pid_lm);
    trq_out_lr=single(trq_dem_lr+(trq_dem_lf-trq_out_lf)+(trq_dem_lm-trq_out_lm));
    trq_out_rm=single(trq_pid_rm);
    trq_out_rr=single(trq_pid_rr);
    trq_out_rf=single(trq_dem_rf+(trq_dem_rm-trq_out_rm)+(trq_dem_rr-trq_out_rr));
    brapre_out_l=single(bra_pre_l+brake_dem);
    brapre_out_r=single(bra_pre_r+brake_dem);
    mode=int8(51);
    
elseif flag_lf==1 && flag_lm==0 && flag_lr==1 && flag_rf==1 && flag_rm==1 && flag_rr==0 %左前-左后 右前-右中 轮滑转
    trq_out_lf=single(trq_pid_lf);
    trq_out_lr=single(trq_pid_lr);
    trq_out_lm=single(trq_dem_lm+(trq_dem_lf-trq_out_lf)+(trq_dem_lr-trq_out_lr));
    trq_out_rf=single(trq_pid_rf);
    trq_out_rm=single(trq_pid_rm);
    trq_out_rr=single(trq_dem_rr+(trq_dem_rf-trq_out_rf)+(trq_dem_rm-trq_out_rm));
    brapre_out_l=single(bra_pre_l+brake_dem);
    brapre_out_r=single(bra_pre_r+brake_dem);
    mode=int8(52);
elseif flag_lf==1 && flag_lm==0 && flag_lr==1 && flag_rf==1 && flag_rm==0 && flag_rr==1 %左前-左后 右前-右后 轮滑转
    trq_out_lf=single(trq_pid_lf);
    trq_out_lr=single(trq_pid_lr);
    trq_out_lm=single(trq_dem_lm+(trq_dem_lf-trq_out_lf)+(trq_dem_lr-trq_out_lr));
    trq_out_rf=single(trq_pid_rf);
    trq_out_rr=single(trq_pid_rr);
    trq_out_rm=single(trq_dem_rm+(trq_dem_rf-trq_out_rf)+(trq_dem_rr-trq_out_rr));
    brapre_out_l=single(bra_pre_l+brake_dem);
    brapre_out_r=single(bra_pre_r+brake_dem);
    mode=int8(53);
elseif flag_lf==1 && flag_lm==0 && flag_lr==1 && flag_rf==0 && flag_rm==1 && flag_rr==1 %左前-左后 右中-右后 轮滑转
    trq_out_lf=single(trq_pid_lf);
    trq_out_lr=single(trq_pid_lr);
    trq_out_lm=single(trq_dem_lm+(trq_dem_lf-trq_out_lf)+(trq_dem_lr-trq_out_lr));
    trq_out_rm=single(trq_pid_rm);
    trq_out_rr=single(trq_pid_rr);
    trq_out_rf=single(trq_dem_rf+(trq_dem_rm-trq_out_rm)+(trq_dem_rr-trq_out_rr));
    brapre_out_l=single(bra_pre_l+brake_dem);
    brapre_out_r=single(bra_pre_r+brake_dem);
    mode=int8(54);
    
elseif flag_lf==0 && flag_lm==1 && flag_lr==1 && flag_rf==1 && flag_rm==1 && flag_rr==0 %左中-左后 右前-右中 轮滑转
    trq_out_lm=single(trq_pid_lm);
    trq_out_lr=single(trq_pid_lr);
    trq_out_lf=single(trq_dem_lf+(trq_dem_lm-trq_out_lm)+(trq_dem_lr-trq_out_lr));
    trq_out_rf=single(trq_pid_rf);
    trq_out_rm=single(trq_pid_rm);
    trq_out_rr=single(trq_dem_rr+(trq_dem_rf-trq_out_rf)+(trq_dem_rm-trq_out_rm));
    brapre_out_l=single(bra_pre_l+brake_dem);
    brapre_out_r=single(bra_pre_r+brake_dem);
    mode=int8(55);
elseif flag_lf==0 && flag_lm==1 && flag_lr==1 && flag_rf==1 && flag_rm==0 && flag_rr==1 %左中-左后 右前-右后 轮滑转
    trq_out_lm=single(trq_pid_lm);
    trq_out_lr=single(trq_pid_lr);
    trq_out_lf=single(trq_dem_lf+(trq_dem_lm-trq_out_lm)+(trq_dem_lr-trq_out_lr));
    trq_out_rf=single(trq_pid_rf);
    trq_out_rr=single(trq_pid_rr);
    trq_out_rm=single(trq_dem_rm+(trq_dem_rf-trq_out_rf)+(trq_dem_rr-trq_out_rr));
    brapre_out_l=single(bra_pre_l+brake_dem);
    brapre_out_r=single(bra_pre_r+brake_dem);
    mode=int8(56);
elseif flag_lf==0 && flag_lm==1 && flag_lr==1 && flag_rf==0 && flag_rm==1 && flag_rr==1 %左中-左后 右中-右后 轮滑转
    trq_out_lm=single(trq_pid_lm);
    trq_out_lr=single(trq_pid_lr);
    trq_out_lf=single(trq_dem_lf+(trq_dem_lm-trq_out_lm)+(trq_dem_lr-trq_out_lr));
    trq_out_rm=single(trq_pid_rm);
    trq_out_rr=single(trq_pid_rr);
    trq_out_rf=single(trq_dem_rf+(trq_dem_rm-trq_out_rm)+(trq_dem_rr-trq_out_rr));
    brapre_out_l=single(bra_pre_l+brake_dem);
    brapre_out_r=single(bra_pre_r+brake_dem);
    mode=int8(57);
    
    
    
    
    
    
    
    
    
    
    
    
    
    
    
    
    
elseif flag_lf==1 && flag_lm==1 && flag_lr==1 && flag_rf==1 && flag_rm==1 && flag_rr==0 %右后轮不划转===================================================5电机滑转
    trq_out_lf=single(trq_pid_lf);
    trq_out_lm=single(trq_pid_lm);
    trq_out_lr=single(trq_pid_lr);
    trq_out_rf=single(trq_pid_rf);
    trq_out_rm=single(trq_pid_rm);
    trq_out_rr=single(trq_dem_rr-((trq_dem_lf-trq_out_lf)+(trq_dem_lm-trq_out_lm)+(trq_dem_lr-trq_out_lr)-(trq_dem_rf-trq_out_rf)-(trq_dem_rm-trq_out_rm)));
    brapre_out_l=single(bra_pre_l+brake_dem);
    brapre_out_r=single(bra_pre_r+brake_dem);
    mode=int8(58);
elseif flag_lf==1 && flag_lm==1 && flag_lr==1 && flag_rf==1 && flag_rm==0 && flag_rr==1 %右中轮不划转
    trq_out_lf=single(trq_pid_lf);
    trq_out_lm=single(trq_pid_lm);
    trq_out_lr=single(trq_pid_lr);
    trq_out_rf=single(trq_pid_rf);
    trq_out_rr=single(trq_pid_rr);
    trq_out_rm=single(trq_dem_rm-((trq_dem_lf-trq_out_lf)+(trq_dem_lm-trq_out_lm)+(trq_dem_lr-trq_out_lr)-(trq_dem_rf-trq_out_rf)-(trq_dem_rr-trq_out_rr)));
    brapre_out_l=single(bra_pre_l+brake_dem);
    brapre_out_r=single(bra_pre_r+brake_dem);
    mode=int8(59);
elseif flag_lf==1 && flag_lm==1 && flag_lr==1 && flag_rf==0 && flag_rm==1 && flag_rr==1 %右前轮不划转
    trq_out_lf=single(trq_pid_lf);
    trq_out_lm=single(trq_pid_lm);
    trq_out_lr=single(trq_pid_lr);
    trq_out_rm=single(trq_pid_rm);
    trq_out_rr=single(trq_pid_rr);
    trq_out_rf=single(trq_dem_rf-((trq_dem_lf-trq_out_lf)+(trq_dem_lm-trq_out_lm)+(trq_dem_lr-trq_out_lr)-(trq_dem_rm-trq_out_rm)-(trq_dem_rr-trq_out_rr)));
    brapre_out_l=single(bra_pre_l+brake_dem);
    brapre_out_r=single(bra_pre_r+brake_dem);
    mode=int8(60);
elseif flag_lf==1 && flag_lm==1 && flag_lr==0 && flag_rf==1 && flag_rm==1 && flag_rr==1 %左后轮不划转===================================================5电机滑转
    trq_out_rf=single(trq_pid_rf);
    trq_out_rm=single(trq_pid_rm);
    trq_out_rr=single(trq_pid_rr);
    trq_out_lf=single(trq_pid_lf);
    trq_out_lm=single(trq_pid_lm);
    trq_out_lr=single(trq_dem_lr-((trq_dem_rf-trq_out_rf)+(trq_dem_rm-trq_out_rm)+(trq_dem_rr-trq_out_rr)-(trq_dem_lf-trq_out_lf)-(trq_dem_lm-trq_out_lm)));
    brapre_out_l=single(bra_pre_l+brake_dem);
    brapre_out_r=single(bra_pre_r+brake_dem);
    mode=int8(61);
elseif flag_lf==1 && flag_lm==0 && flag_lr==1 && flag_rf==1 && flag_rm==1 && flag_rr==1 %左中轮不划转
    trq_out_rf=single(trq_pid_rf);
    trq_out_rm=single(trq_pid_rm);
    trq_out_rr=single(trq_pid_rr);
    trq_out_lf=single(trq_pid_lf);
    trq_out_lr=single(trq_pid_lr);
    trq_out_lm=single(trq_dem_lm-((trq_dem_rf-trq_out_rf)+(trq_dem_rm-trq_out_rm)+(trq_dem_rr-trq_out_rr)-(trq_dem_lf-trq_out_lf)-(trq_dem_lr-trq_out_lr)));
    brapre_out_l=single(bra_pre_l+brake_dem);
    brapre_out_r=single(bra_pre_r+brake_dem);
    mode=int8(62);
elseif flag_lf==0 && flag_lm==1 && flag_lr==1 && flag_rf==1 && flag_rm==1 && flag_rr==1 %左前轮不划转
    trq_out_rf=single(trq_pid_rf);
    trq_out_rm=single(trq_pid_rm);
    trq_out_rr=single(trq_pid_rr);
    trq_out_lm=single(trq_pid_lm);
    trq_out_lr=single(trq_pid_lr);
    trq_out_lf=single(trq_dem_lf-((trq_dem_rf-trq_out_rf)+(trq_dem_rm-trq_out_rm)+(trq_dem_rr-trq_out_rr)-(trq_dem_lm-trq_out_lm)-(trq_dem_lr-trq_out_lr)));
    brapre_out_l=single(bra_pre_l+brake_dem);
    brapre_out_r=single(bra_pre_r+brake_dem);
    mode=int8(63);
    
    
    
    
    
    
    
    
    
    
    
    
    
else
    %     flag_lf==1 && flag_lm==1 && flag_lr==1 && flag_rf==1 && flag_rm==1 && flag_rr==1 %===================================================6电机滑转
    trq_out_lf=single(trq_pid_lf);
    trq_out_lm=single(trq_pid_lm);
    trq_out_lr=single(trq_pid_lr);
    trq_out_rf=single(trq_pid_rf);
    trq_out_rm=single(trq_pid_rm);
    trq_out_rr=single(trq_pid_rr);
    trqcha=(trq_dem_lf-trq_out_lf)+(trq_dem_lm-trq_out_lm)+(trq_dem_lr-trq_out_lr)-(trq_dem_rf-trq_out_rf)-(trq_dem_rm-trq_out_rm)-(trq_dem_rr-trq_out_rr);
    if trqcha>=0
        trq_out_rf=trq_pid_rf-trqcha/3;
        trq_out_rm=trq_pid_rm-trqcha/3;
        trq_out_rr=trq_pid_rr-trqcha/3;
    else
        trq_out_lf=trq_pid_lf+trqcha/3;
        trq_out_lm=trq_pid_lm+trqcha/3;
        trq_out_lr=trq_pid_lr+trqcha/3;
    end
    brapre_out_l=single(bra_pre_l+brake_dem);
    brapre_out_r=single(bra_pre_r+brake_dem);
    mode=int8(64);
end



trq_out_lf=single(trq_out_lf);
trq_out_lm=single(trq_out_lm);
trq_out_lr=single(trq_out_lr);
trq_out_rf=single(trq_out_rf);
trq_out_rm=single(trq_out_rm);
trq_out_rr=single(trq_out_rr);
brapre_out_l=single(brapre_out_l);
brapre_out_r=single(brapre_out_r);
end
